simulink model "scheme4"  (R2024a)
settings: Solver=VariableStepAuto  StartTime=0.0  StopTime=60  RelTol=1e-6
undefined symbols (not defined in the file): func, k
settings Model: Creator=alexivanov  LastModifiedBy=alexivanov

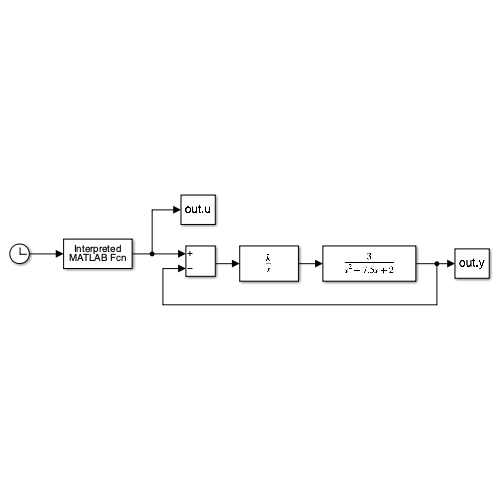
[thumbnail: Simulink's stored preview of the top-level diagram]
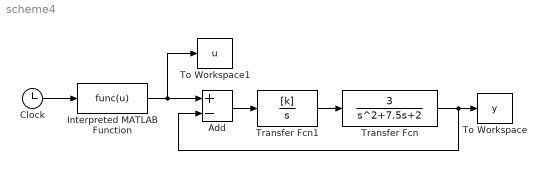
== system scheme4 ==
  Add : Sum  Inputs=+-
  Clock : Clock
  Interpreted MATLAB Function : MATLABFcn  MATLABFcn=func(u)
  To Workspace : ToWorkspace  VariableName=y  SaveFormat=Timeseries  SampleTime=-1
  To Workspace1 : ToWorkspace  VariableName=u  SaveFormat=Timeseries  SampleTime=-1
  Transfer Fcn : TransferFcn  Numerator=[3]  Denominator=[1 7.5 2]
  Transfer Fcn1 : TransferFcn  Numerator=[k]  Denominator=[1, 0]
  wires:
  Clock/1 -> Interpreted MATLAB Function/1
  Transfer Fcn1/1 -> Transfer Fcn/1
  Add/1 -> Transfer Fcn1/1
  Interpreted MATLAB Function/1 -> To Workspace1/1, Add/1
  Transfer Fcn/1 -> Add/2, To Workspace/1
